simulink model "modeling"  (R2023a)
settings: Solver=VariableStepAuto  StartTime=0.0  StopTime=1800  RelTol=1e-3
undefined symbols (not defined in the file): Ion, Lithium
libraries: spsBatteryLib x12, spsControlledVoltageSourceLib x1, autolibshared x1, spsVoltageMeasurementLib x1, sps_lib x1
settings Model: Creator=DELL  LastModifiedBy=DELL

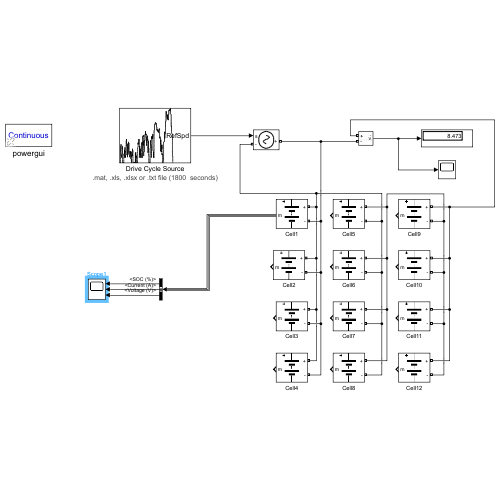
[thumbnail: Simulink's stored preview of the top-level diagram]
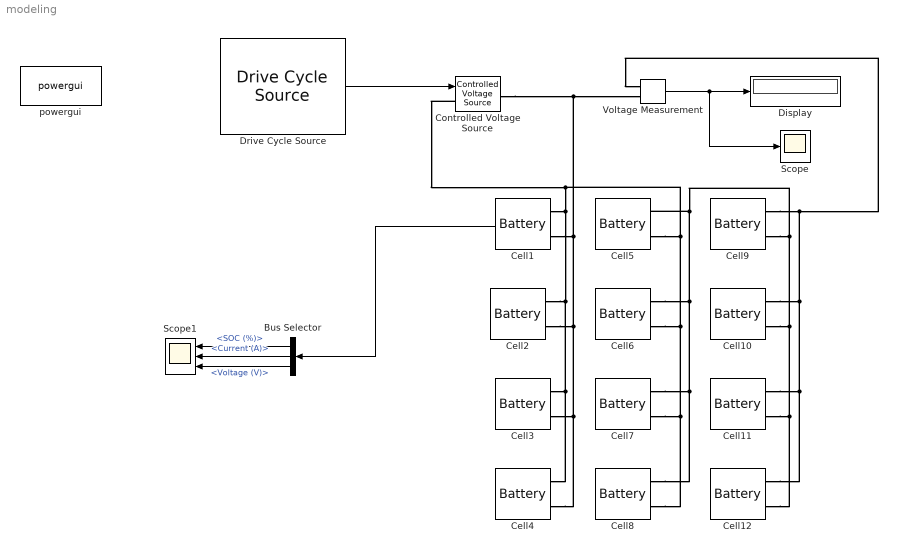
== system modeling ==
  Bus Selector : BusSelector  OutputSignals=SOC (%),Current (A),Voltage (V)
  Cell{1..12} (12 alike) : spsBatteryLib/Battery  BatType=Lithium-Ion  ShowTempParam=off  ThermalPreset=no  ShowAgeParam=off  NomV=3.7  NomQ=3  SOC=100  Batt_Tr=30  PresetModel=off  MaxQ=2.6  MinV=3  FullV=4.2  Dis_rate=0.52  R=0.07  Normal_OP=2.55  expZone="[4      0.4]"  current=[0.52 1.3 2.6]  Units=Ampere-hour  Tci=20  NomT=20  T2=-30  MaxQ2=4.8  FullV2=7.1  Normal_OP2=5.655  expZone2="[6.58           1]"  Rca=0.6  ti=2000  Dp=0  Neq0=0  Tsim=1e6  Ta1=25  Qeol=5.4*0.9  Reol=0.013333*1.2  Char_age=[2.3478, 3]  Dis_age=[2.3478, 10]  N1=1500  N2=10500  N3=1000  N4=1400  Ta2=45  N5=950
  Controlled Voltage Source : spsControlledVoltageSourceLib/Controlled Voltage Source  Initialize=on  Source_Type=DC  Amplitude=0  Phase=0  Frequency=0  Measurements=None
  Display : Display
  Drive Cycle Source : autolibshared/Drive Cycle Source  cycleVar=.mat, .xls, .xlsx or .txt file  fileVar=C:\Users\DELL\Desktop\Summer Project\BMS\battery modeling\WLTC_DC_Datasheet.xlsx  tfinal="1800  seconds"  cycleRepeat=off  outAccPort=off  outGearPort=off  gearList=No gear data  t_wot1=5  xdot_woto=0  xdot_wot1=30  t_wot2=20  xdot_wot2=0  t_wotend=30  srcUnit=m/s  outUnit=m/s  srcAccUnit=m/s/s  outAccUnit=m/s^2  dt=0  aMode=1  faultOption=off  velBnd=2  velBndUnit=mph  inUnit=m/s  timeBnd=1  failOption=off  stopSim=off  maxFaultCnt=10  maxFaultTime=2  maxTotFaultTime=15  traceOption=off  dtTrace=1  traceWindow=10  lastDCname=Custom Data Set  lastOutUnit=mph  lastDT=0  lastTB=1  lastSB=2  forceCalcBound=off
  Scope : Scope
  Scope1 : Scope  NumInputPorts=3
  Voltage Measurement : spsVoltageMeasurementLib/Voltage Measurement  PhasorSimulation=off  OutputType=Complex  PSBequivalent=0
  powergui : sps_lib/powergui  Priority=1  SimulationMode=Continuous  SampleTime=50e-6  frequency=60  Iterations=50  frequencyindice=0  Pbase=100e6  ErrMax=1e-4  UnitsV=kV  UnitsW=MW  buscounter=0  FunctionMessages=off  echomessages=off  EnableUseOfTLC=off  CurrentSourceSwitches=off  DisableSnubberDevices=off  DisableRonSwitches=off  DisableVfSwitches=off  DisplayEquations=off  AutomaticDiscreteSolvers=off  SolverType=Tustin/Backward Euler (TBE)  Interpol=off  ExternalGateDelay=off  methode=off  Ts=100  x0status=blocks  SPID=on  SwTol=0  HookPort=off  NonlinearTolerance=1e-4  nMaxIteration=100  ContinueOnMaxIteration=off  RestoreLinks=warning  ResistiveCurrentMeasurement=off  Frange=[0:2:500]  Ylog=off  Xlog=on  ShowGrid=off  save=off  variable=ZData  structure=0  ZoomFFT=off  StartTime=0.0  cycles=1  DisplayStyle=1  fundamental=60  FreqAxis=off  MaxFrequency=1000  frequencyindicesteady=1  RmsSteady=1  display=off
  wires:
  Drive Cycle Source/1 -> Controlled Voltage Source/1
  Voltage Measurement/1 -> Scope/1, Display/1
  Cell1/1 -> Bus Selector/1
  Bus Selector/1 -> Scope1/1  "<SOC (%)>"
  Bus Selector/2 -> Scope1/2  "<Current (A)>"
  Bus Selector/3 -> Scope1/3  "<Voltage (V)>"
  connections:
  Cell1/LConn1 -- Cell5/LConn2 -- Cell6/LConn2 -- Cell8/LConn2 -- Cell7/LConn2 -- Controlled Voltage Source/LConn1 -- Cell4/LConn1 -- Cell3/LConn1 -- Cell2/LConn1
  Cell6/LConn1 -- Cell8/LConn1 -- Cell7/LConn1 -- Cell12/LConn2 -- Cell11/LConn2 -- Cell10/LConn2 -- Cell9/LConn2 -- Cell5/LConn1
  Cell4/LConn2 -- Cell3/LConn2 -- Cell2/LConn2 -- Controlled Voltage Source/RConn1 -- Voltage Measurement/LConn2 -- Cell1/LConn2
  Cell9/LConn1 -- Cell12/LConn1 -- Cell11/LConn1 -- Cell10/LConn1 -- Voltage Measurement/LConn1
